simulink model "untitled2_1"  (R2018b)
settings: Solver=VariableStepAuto  StartTime=0.0  StopTime=10  RelTol=1e-3
libraries: dsparch4 x1
settings Model: Creator=nhat  LastModifiedBy=nhat

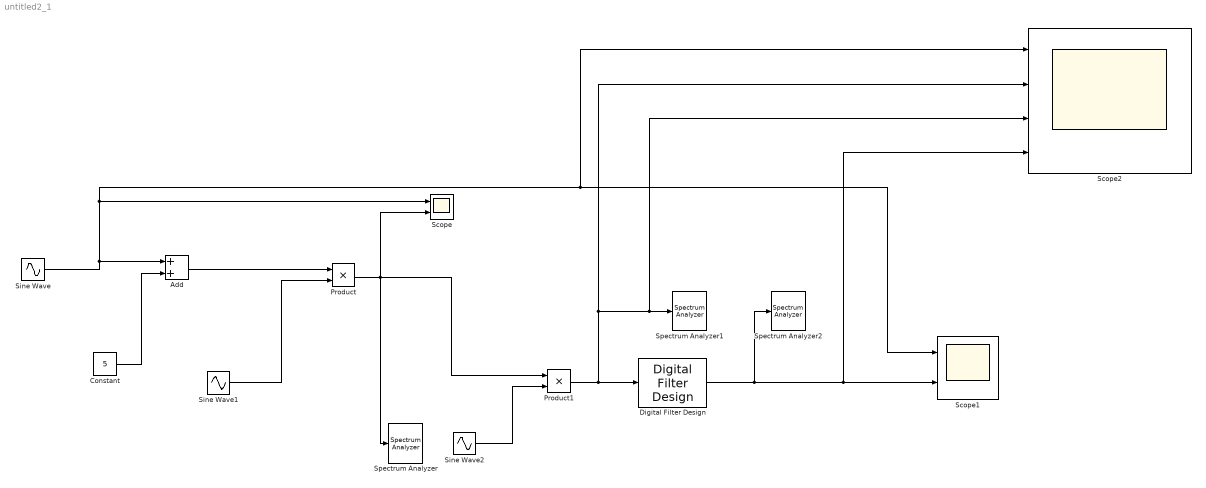
== system untitled2_1 ==
  Add : Sum
  Constant : Constant  Value=5
  Digital Filter Design : dsparch4/Digital Filter Design  mwdsp_browser_bugfix_var=off
  Product : Product
  Product1 : Product
  Scope : Scope  NumInputPorts=2
  Scope1 : Scope  NumInputPorts=2
  Scope2 : Scope  NumInputPorts=4
  Sine Wave : Sin  Amplitude=0.5  Frequency=200*2*pi  SampleTime=1/40000
  Sine Wave1 : Sin  Frequency=5000*2*pi  SampleTime=1/40000
  Sine Wave2 : Sin  Frequency=5000*2*pi  SampleTime=1/40000
  Spectrum Analyzer : SpectrumAnalyzer
  Spectrum Analyzer1 : SpectrumAnalyzer
  Spectrum Analyzer2 : SpectrumAnalyzer
  wires:
  Sine Wave2/1 -> Product1/2
  Product1/1 -> Scope2/2, Spectrum Analyzer1/1, Scope2/3, Digital Filter Design/1
  Digital Filter Design/1 -> Scope2/4, Scope1/2, Spectrum Analyzer2/1
  Sine Wave/1 -> Add/1, Scope2/1, Scope1/1, Scope/1
  Product/1 -> Scope/2, Spectrum Analyzer/1, Product1/1
  Add/1 -> Product/1
  Constant/1 -> Add/2
  Sine Wave1/1 -> Product/2
